simulink model "ESC_Model"  (R2025a)
settings: Solver=VariableStepAuto  StartTime=0.0  StopTime=10.0  RelTol=1e-3
settings Model: Creator=Ayush_S  LastModifiedBy=Ayush_S

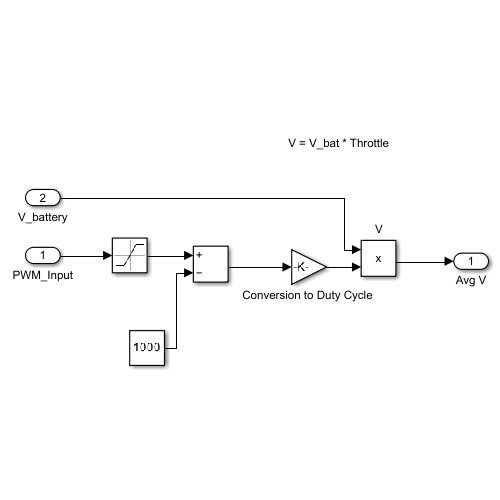
[thumbnail: Simulink's stored preview of the top-level diagram]
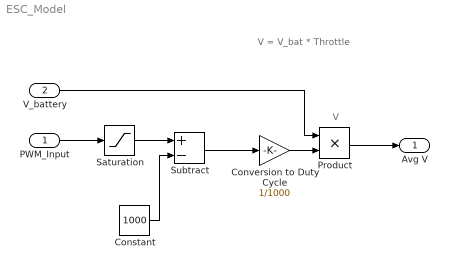
== system ESC_Model ==
  note: V = V_bat * Throttle
  note: V
  PWM_Input : Inport
  V_battery : Inport  Port=2
  Constant : Constant  Value=1000
  "Conversion to Duty Cycle " : Gain  Gain=1/1000
  Product : Product
  Saturation : Saturate  UpperLimit=2000  LowerLimit=1000
  Subtract : Sum  Inputs=+-
  Avg V : Outport
  wires:
  Constant/1 -> Subtract/2
  "Conversion to Duty Cycle "/1 -> Product/2
  V_battery/1 -> Product/1
  Saturation/1 -> Subtract/1
  PWM_Input/1 -> Saturation/1
  Subtract/1 -> "Conversion to Duty Cycle "/1
  Product/1 -> Avg V/1
